simulink model "New_SPD_For_Test"  (R2014b)
settings: Solver=FixedStepDiscrete  StartTime=0.0  StopTime=200  RelTol=1e-3
libraries: BlockLib x21, dspsrcs4 x1
settings Model: Creator=Alexander  LastModifiedBy=kunalmenda

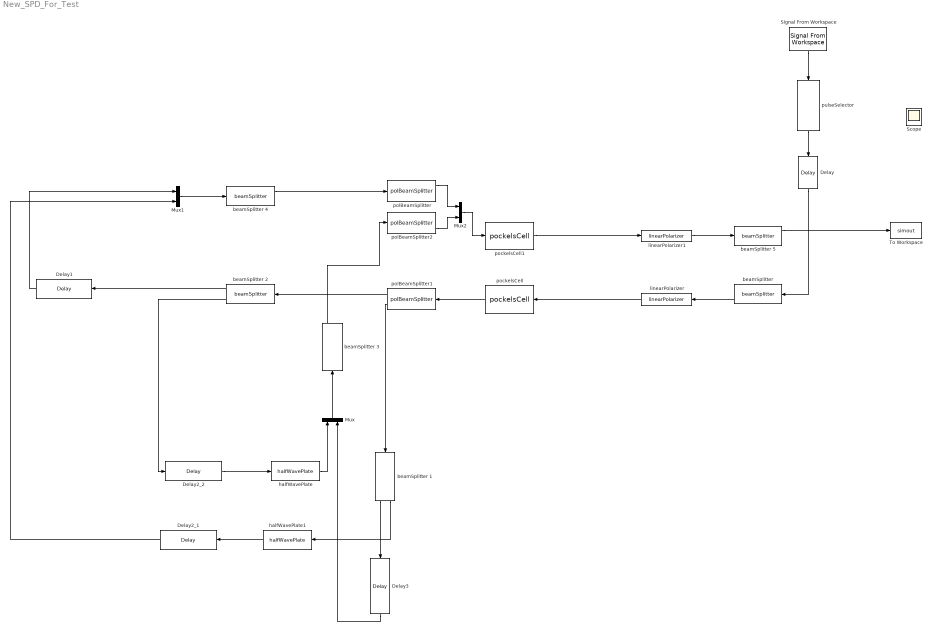
== system New_SPD_For_Test ==
  Delay : BlockLib/Delay  DelayAmt=3e-9
  Delay1 : BlockLib/Delay  DelayAmt=10e-9
  Delay2_1 : BlockLib/Delay  DelayAmt=14.33e-9
  Delay2_2 : BlockLib/Delay  DelayAmt=14.33e-9
  Delay3 : BlockLib/Delay  DelayAmt=18.66e-9
  Mux : Mux  Inputs=2
  Mux1 : Mux  Inputs=2
  Mux2 : Mux  Inputs=2
  Scope : Scope
  Signal From Workspace : dspsrcs4/Signal From Workspace  X=inputsignal  Ts=1  nsamps=1  OutputAfterFinalValue=Setting to zero  ignoreOrWarnInputAndFrameLengths=off
  To Workspace : ToWorkspace  VariableName=simout  SaveFormat=Timeseries  SampleTime=-1
  beamSplitter {,1..5} (6 alike) : BlockLib/beamSplitter 
  halfWavePlate : BlockLib/halfWavePlate  AxisAngle=pi/4
  halfWavePlate1 : BlockLib/halfWavePlate  AxisAngle=pi/4
  linearPolarizer : BlockLib/linearPolarizer  AxisAngle=pi/2
  linearPolarizer1 : BlockLib/linearPolarizer  AxisAngle=pi/2
  pockelsCell : BlockLib/pockelsCell  OutputDimensions=1  AxisAngle=pi/4  PCID=PC2.ID
  pockelsCell1 : BlockLib/pockelsCell  OutputDimensions=4  AxisAngle=pi/4  PCID=PC2.ID
  polBeamSplitter : BlockLib/polBeamSplitter
  polBeamSplitter1 : BlockLib/polBeamSplitter
  polBeamSplitter2 : BlockLib/polBeamSplitter
  pulseSelector : BlockLib/pulseSelector  OutputDimensions=1  PCID=PC1.ID
  wires:
  polBeamSplitter1/2 -> beamSplitter 1/1
  polBeamSplitter1/1 -> beamSplitter 2/1
  beamSplitter 2/1 -> Delay1/1
  beamSplitter 1/1 -> Delay3/1
  beamSplitter 1/2 -> halfWavePlate1/1
  halfWavePlate1/1 -> Delay2_1/1
  Delay2_1/1 -> Mux1/2
  Delay3/1 -> Mux/2
  Mux/1 -> beamSplitter 3/1
  halfWavePlate/1 -> Mux/1
  Mux1/1 -> beamSplitter 4/1
  Delay1/1 -> Mux1/1
  beamSplitter 4/1 -> polBeamSplitter/1
  beamSplitter 3/1 -> polBeamSplitter2/1
  Delay2_2/1 -> halfWavePlate/1
  pockelsCell1/1 -> linearPolarizer1/1
  linearPolarizer1/1 -> beamSplitter 5/1
  "beamSplitter "/2 -> linearPolarizer/1
  beamSplitter 2/2 -> Delay2_2/1
  pockelsCell/1 -> polBeamSplitter1/1
  polBeamSplitter/1 -> Mux2/1
  polBeamSplitter2/2 -> Mux2/2
  Mux2/1 -> pockelsCell1/1
  Signal From Workspace/1 -> pulseSelector/1
  beamSplitter 5/1 -> To Workspace/1
  pulseSelector/1 -> Delay/1
  linearPolarizer/1 -> pockelsCell/1
  Delay/1 -> "beamSplitter "/1
